simulink model "rigid_body_fdyn_rotmat_test_nocom"  (Simulink 8.5)
settings: Solver=ode4  StartTime=0.0  StopTime=10.0  FixedStep=1.000000e-04  RelTol=1e-3
undefined symbols (not defined in the file or in its folder): g_W, I_B_C, m
libraries: lib_rigid_body_dynamics x4
settings Model: Creator=schappler  LastModifiedBy=schappler
settings DataIOCC: LimitDataPoints=off  SaveFormat=StructureWithTime  SignalLoggingSaveFormat=Dataset
settings OptimizationCC: ExpressionDepthLimit=128
settings DebuggingCC: UnderspecifiedInitializationDetection=Simplified  MergeDetectMultiDrivingBlocksExec=error  FcnCallInpInsideContextMsg=EnableAllAsError  StateNameClashWarn=none
settings GRTTargetCC: CombineOutputUpdateFcns=on  GRTInterface=off

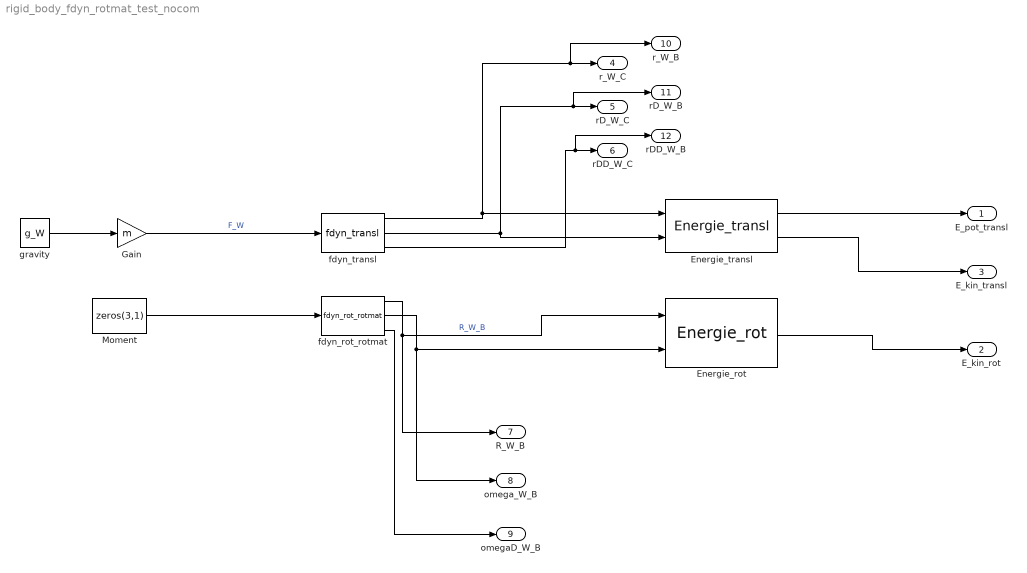
== system rigid_body_fdyn_rotmat_test_nocom ==
  Energie_rot : lib_rigid_body_dynamics/Energie_rot  I_B_C=I_B_C
  Energie_transl : lib_rigid_body_dynamics/Energie_transl  m=m  g_W=g_W
  Gain : Gain  Gain=m
  Moment : Constant  Value=zeros(3,1)
  fdyn_rot_rotmat : lib_rigid_body_dynamics/fdyn_rot_rotmat  I=I_B_C  R_0E_t0=R_W_B_t0  omega0_t0=omega0_t0
  fdyn_transl : lib_rigid_body_dynamics/fdyn_transl  m=m  r0=r0  rD0=rD0
  gravity : Constant  Value=g_W
  E_pot_transl : Outport
  E_kin_rot : Outport  Port=2
  E_kin_transl : Outport  Port=3
  r_W_C : Outport  Port=4
  rD_W_C : Outport  Port=5
  rDD_W_C : Outport  Port=6
  R_W_B : Outport  Port=7
  omega_W_B : Outport  Port=8
  omegaD_W_B : Outport  Port=9
  r_W_B : Outport  Port=10
  rD_W_B : Outport  Port=11
  rDD_W_B : Outport  Port=12
  wires:
  gravity/1 -> Gain/1
  fdyn_rot_rotmat/1 -> Energie_rot/1, R_W_B/1  "R_W_B"
  Gain/1 -> fdyn_transl/1  "F_W"
  fdyn_transl/1 -> Energie_transl/1, r_W_B/1, r_W_C/1
  fdyn_transl/2 -> Energie_transl/2, rD_W_B/1, rD_W_C/1
  fdyn_rot_rotmat/2 -> Energie_rot/2, omega_W_B/1
  fdyn_transl/3 -> rDD_W_B/1, rDD_W_C/1
  fdyn_rot_rotmat/3 -> omegaD_W_B/1
  Moment/1 -> fdyn_rot_rotmat/1
  Energie_transl/1 -> E_pot_transl/1
  Energie_transl/2 -> E_kin_transl/1
  Energie_rot/1 -> E_kin_rot/1
